simulink model "XMC_FFT2D_HDL_AIE"  (R2020a)
settings: Solver=FixedStepDiscrete  StartTime=0.0  StopTime=256*256*2  RelTol=1e-3
PreLoadFcn:
  | MRIDemo_PreloadFcn;
  | 
  | % configure hardware specifics information
  | clock_frequency = 150e6;
  | 
  | % corner bender info
  | clk = clock_frequency; %Hz
  | Tclk = 1/clk;
  | L2M = 8; % L2M=log2(M)
  | L2N = 8; % L2N=log2(N)
  | M = 2^L2M;
  | N = 2^L2N;
  | SSR = 1;
InitFcn:
  | xlEvaluateHDLBlocks('XMC_FFT2D_HDL_AIE')
undefined symbols (not defined in the file): c, gray, S, vsva2197, xcvc1902
libraries: xbsIndex_r4 x132, ModelComposer x6, dspxfrm3 x2, dspsrcs4 x2
(part 1 of 2)
settings Model: PauseTimes=256*254  SnapshotBufferSize=1000  SnapshotInterval=1  Creator=mmi  LastModifiedBy=viswanad
settings DataIOCC: ReturnWorkspaceOutputs=off
settings DebuggingCC: ArithmeticOperatorsInVariantConditions=warning
settings SFSimCC: SimUseLocalCustomCode=off  CustomCodeUndefinedFunction=UseInterfaceOnly
settings RTWCC: RTWUseLocalCustomCode=off

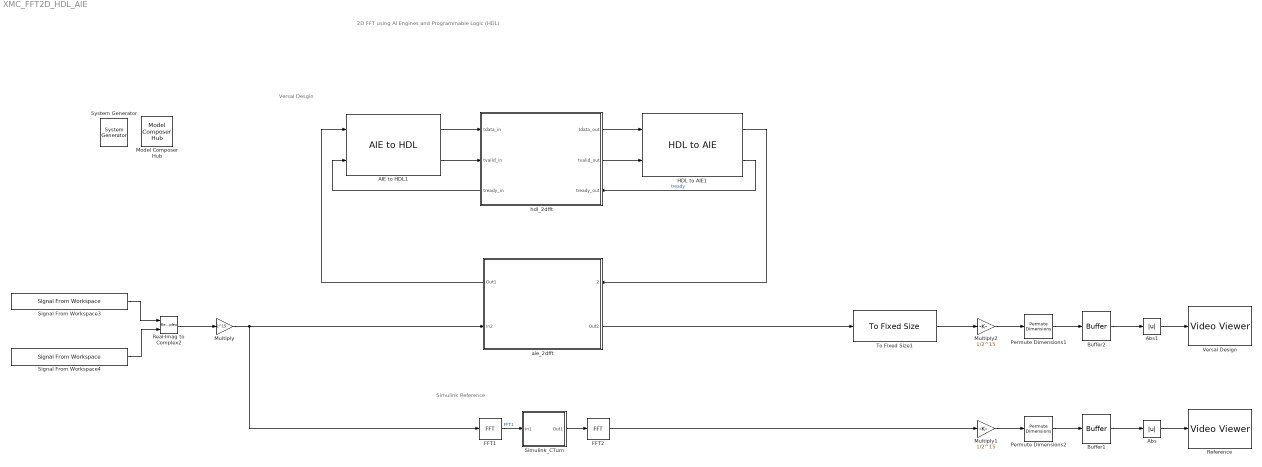
== system XMC_FFT2D_HDL_AIE ==
  note: Versal Desgin
  note: Simulink Reference
  note: 2D FFT using
      | AI Engines and Programmable Logic (HDL)
  " System Generator" : xbsIndex_r4/ System Generator  Tag=genX  xilinxfamily=versalaicore  part=xcvc1902  speed=-3HP-e-S  package=viva1596  synthesis_tool=Vivado  clock_wrapper=Clock Enables  directory=./netlist  proj_type=Vivado  Synth_file=Vivado Synthesis Defaults  Impl_file=Vivado Implementation Defaults  testbench=off  simulink_period=1  sysclk_period=4  dcm_input_clock_period=10  incr_netlist=off  trim_vbits=Everywhere in SubSystem  dbl_ovrd=According to Block Masks  core_generation=According to Block Masks  run_coregen=off  deprecated_control=off  eval_field=0  block_type=sysgen
  AIE to HDL1 : ModelComposer/AIE to HDL  OutDataType=uint32  OutSampleTime=1
      link override AIE to HDL_tready: inherit_from_input=on  hdl_port=on  rows=1  columns=1  UseAsDAC=off  DACChannel='1'  interface=None  automatic_assignment=on  address_offset=hex2dec('00')  intf_name=''  intf_description=''  timing_constraint=None  locs_specified=off  LOCs={}  io_standard={}
      link override AIE to HDL_tready: infoedit="Gateway out block.  Converts Xilinx fixed-point or floating-point type inputs into ouputs of type Simulink integer, single, double, or fixed-point.<br><br>Hardware notes:  In hardware these blocks become top level output ports or are discarded, depending on how they are configured."
  Abs : Abs
  Abs1 : Abs
  Buffer1 : Buffer  N=256  OutputFrames=off
  Buffer2 : Buffer  N=256  OutputFrames=off
  FFT1 : dspxfrm3/FFT  FFTImplementation=Auto  CompMethod=Table lookup  TableOpt=NEW  TableOptActive=Speed  BitRevOrder=off  Normalize=off  InheritFFTLength=on  FFTLength=64  WrapInput=on  roundingMode=Floor  overflowMode=off  firstCoeffDataTypeStr=Inherit: Same word length as input  firstCoeffLastDataTypeStr=Inherit: Same word length as input  prodOutputMode=Binary point scaling  prodOutputWordLength=32  prodOutputFracLength=0  prodOutputDataTypeStr=fixdt(1,32,0)  prodOutputLastDataTypeStr=fixdt(1,32,0)  accumMode=Binary point scaling  accumWordLength=48  accumFracLength=0  accumDataTypeStr=fixdt(1,48,0)  accumLastDataTypeStr=fixdt(1,48,0)  outputMode=Binary point scaling  outputWordLength=16  outputFracLength=0  outputDataTypeStr=fixdt(1,16,0)  outputMin=[]  outputMax=[]  outputLastDataTypeStr=fixdt(1,16,0)
  FFT2 : dspxfrm3/FFT  FFTImplementation=Auto  CompMethod=Table lookup  TableOpt=NEW  TableOptActive=Speed  BitRevOrder=off  Normalize=off  InheritFFTLength=on  FFTLength=64  WrapInput=on  roundingMode=Floor  overflowMode=off  firstCoeffDataTypeStr=Inherit: Same word length as input  firstCoeffLastDataTypeStr=Inherit: Same word length as input  prodOutputMode=Binary point scaling  prodOutputWordLength=32  prodOutputFracLength=0  prodOutputDataTypeStr=fixdt(1,32,0)  prodOutputLastDataTypeStr=fixdt(1,32,0)  accumMode=Binary point scaling  accumWordLength=48  accumFracLength=0  accumDataTypeStr=fixdt(1,48,0)  accumLastDataTypeStr=fixdt(1,48,0)  outputMode=Binary point scaling  outputWordLength=16  outputFracLength=0  outputDataTypeStr=fixdt(1,16,0)  outputMin=[]  outputMax=[]  outputLastDataTypeStr=fixdt(1,16,0)
  HDL to AIE1 : ModelComposer/HDL to AIE  OutDataType=int16 (c)  OutSampleTime=1  SamplesPerFrame=256  TreadySampleTime=1
  Model Composer Hub : ModelComposer/Model Composer Hub  CodeGeneration=off  SubsystemName=aie_2dfft  TargetDirectory=./code  ExportType=AI Engines  IpVendor=xilinx.com  IpLibrary=hls  IpVersion=1.0  IpHWLanguage=Verilog  AieCompilerOptions={}  CreateTestbench=on  TestbenchStackSize=10  RunAieSim=on  AieSimTimeout=50000  RunAieSimProfiling=off  LaunchVitisAnalyzer=off  PlotOutput=off  RunX86Sim=off  X86SimTimeout=10  PlatformType=Not Specified  ProjDevice=xcvc1902-vsva2197-2MP-e-S  ProjDevicePart=xcvc1902-vsva2197-2MP-e-S  SamplePeriod=-1  ClockFrequency=150  DataPathParallelism=1
  Multiply : Gain  Gain=2^15  OutDataTypeStr=int16
  Multiply1 : Gain  Gain=1/2^15  OutDataTypeStr=single
  Multiply2 : Gain  Gain=1/2^15  OutDataTypeStr=single
  Permute Dimensions1 : PermuteDimensions
  Permute Dimensions2 : PermuteDimensions
  Real-Imag to Complex2 : RealImagToComplex
  Reference : VideoViewer  Description=Simulink MRI Display  colormapValue=gray(256)  FigPos=[1258 828 663 270]
  Signal From Workspace3 : dspsrcs4/Signal From Workspace  X=MRIDemo_data_real_channel  Ts=1  nsamps=256  OutputAfterFinalValue=Setting to zero  ignoreOrWarnInputAndFrameLengths=off  OutputFrames=off
  Signal From Workspace4 : dspsrcs4/Signal From Workspace  X=MRIDemo_data_imag_channel  Ts=1  nsamps=256  OutputAfterFinalValue=Setting to zero  ignoreOrWarnInputAndFrameLengths=off  OutputFrames=off
  Simulink_CTurn : Subsystem
  To Fixed Size1 : ModelComposer/To Fixed Size  OutputSize=256  HasStatusOutput=off
  Versal Design : VideoViewer  Description=Simulink MRI Display  colormapValue=gray(256)  FigPos=[720 707 653 277]
  aie_2dfft : Subsystem
      settings: PortSchema="{\"entries\":[{\"content\":{\"sides\":[{\"content\":{\"connectorIds\":[\"Out2\",\"In1\"]},\"type\":\"ConnectorPlacement.EquallySpacedRectSide\",\"uuid\":\"ba116f73-e116-40b3-b2e5-304cba4df7e1\"},{\"content\":{\"connectorIds\":[\"In2\",\"Out1\"],\"side\":\"RIGHT\"},\"type\":\"ConnectorPlacement.EquallySpacedRectSide\",\"uuid\":\"f8ace37c-ffb0-4f56-a1b3-7eeef7565cfd\"},{\"content\":{\"connectorIds\":[],\"side\":\"TOP\"},\"type\":\"ConnectorPlacement.EquallySpacedRectSide\",\"uuid\":\"698d2e0a-1e8b-402b-bc99-cd34e1f9cd41\"}]},\"type\":\"ConnectorPlacement.EquallySpacedConnector\",\"uuid\":\"c9271cff-0d68-4ac4-bc57-5327e013a37e\"}],\"packageUris\":[\"http://schema.mathworks.com/mf0/Connector/R2020b\"],\"version\":\"1.0\"}"
  hdl_2dfft : Subsystem
      settings: PortSchema="{\"entries\":[{\"content\":{\"sides\":[{\"content\":{\"connectorIds\":[\"In1\",\"In2\",\"Out3\"]},\"type\":\"ConnectorPlacement.EquallySpacedRectSide\",\"uuid\":\"096cfc4a-45cf-495e-9dad-5ec39c034de1\"},{\"content\":{\"connectorIds\":[\"Out1\",\"Out2\",\"In3\"],\"side\":\"RIGHT\"},\"type\":\"ConnectorPlacement.EquallySpacedRectSide\",\"uuid\":\"c2f58c53-17c1-4e0f-8fe6-4ca31b4ae7e7\"},{\"content\":{\"connectorIds\":[],\"side\":\"TOP\"},\"type\":\"ConnectorPlacement.EquallySpacedRectSide\",\"uuid\":\"fc0a0e48-62d9-4bc4-85b8-28883543f418\"}]},\"type\":\"ConnectorPlacement.EquallySpacedConnector\",\"uuid\":\"4d40c623-5fa9-4077-a912-8400e8a8f04d\"}],\"packageUris\":[\"http://schema.mathworks.com/mf0/Connector/R2020b\"],\"version\":\"1.0\"}"
  wires:
  HDL to AIE1/1 -> aie_2dfft/2(" ")
  Real-Imag to Complex2/1 -> Multiply/1
  Signal From Workspace3/1 -> Real-Imag to Complex2/1
  Signal From Workspace4/1 -> Real-Imag to Complex2/2
  hdl_2dfft/2(tvalid_out) -> HDL to AIE1/2
  hdl_2dfft/1(tdata_out) -> HDL to AIE1/1
  AIE to HDL1/2 -> hdl_2dfft/2(tvalid_in)
  AIE to HDL1/1 -> hdl_2dfft/1(tdata_in)
  aie_2dfft/2(Out1) -> AIE to HDL1/1
  HDL to AIE1/2 -> hdl_2dfft/3(tready_out)  "tready"
  hdl_2dfft/3(tready_in) -> AIE to HDL1/2
  Multiply1/1 -> Permute Dimensions2/1
  Abs/1 -> Reference/1
  Permute Dimensions2/1 -> Buffer1/1
  Buffer1/1 -> Abs/1
  Multiply/1 -> FFT1/1, aie_2dfft/1(In2)
  FFT1/1 -> Simulink_CTurn/1(In1)  "FFT1"
  FFT2/1 -> Multiply1/1
  Simulink_CTurn/1(Out1) -> FFT2/1
  Abs1/1 -> Versal Design/1
  Buffer2/1 -> Abs1/1
  Permute Dimensions1/1 -> Buffer2/1
  Multiply2/1 -> Permute Dimensions1/1
  aie_2dfft/1(Out2) -> To Fixed Size1/1
  To Fixed Size1/1 -> Multiply2/1

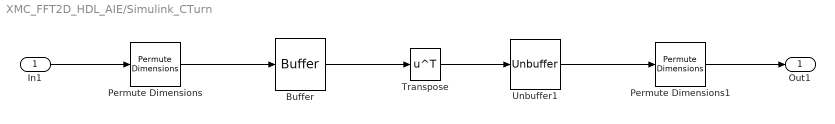
== system XMC_FFT2D_HDL_AIE/Simulink_CTurn ==
  In1 : Inport
  Buffer : Buffer  N=256  OutputFrames=off
  Permute Dimensions : PermuteDimensions
  Permute Dimensions1 : PermuteDimensions
  Transpose : Math  Operator=transpose  SignedPower=on  SaturateOnIntegerOverflow=on
  Unbuffer1 : Unbuffer
  Out1 : Outport  VectorParamsAs1DForOutWhenUnconnected=off
  wires:
  Permute Dimensions/1 -> Buffer/1
  Transpose/1 -> Unbuffer1/1
  Buffer/1 -> Transpose/1
  In1/1 -> Permute Dimensions/1
  Unbuffer1/1 -> Permute Dimensions1/1
  Permute Dimensions1/1 -> Out1/1

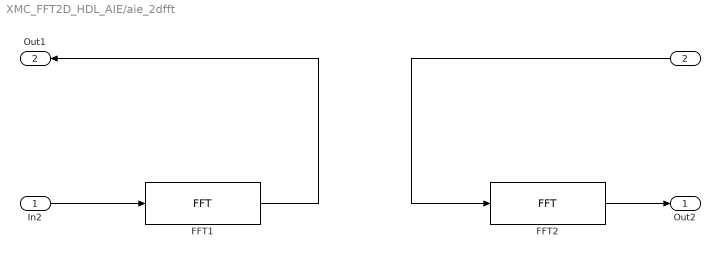
== system XMC_FFT2D_HDL_AIE/aie_2dfft ==
  In2 : Inport
  " " : Inport  Port=2
  FFT1 : ModelComposer/FFT  data_type=cint16  point_size=256  casc_length=1  shift_val=0  spec=meta_data_hl_fft.json
  FFT2 : ModelComposer/FFT  data_type=cint16  point_size=256  casc_length=1  shift_val=0  spec=meta_data_hl_fft.json
  Out2 : Outport
  Out1 : Outport  Port=2
  wires:
  FFT2/1 -> Out2/1
  " "/1 -> FFT2/1
  FFT1/1 -> Out1/1
  In2/1 -> FFT1/1

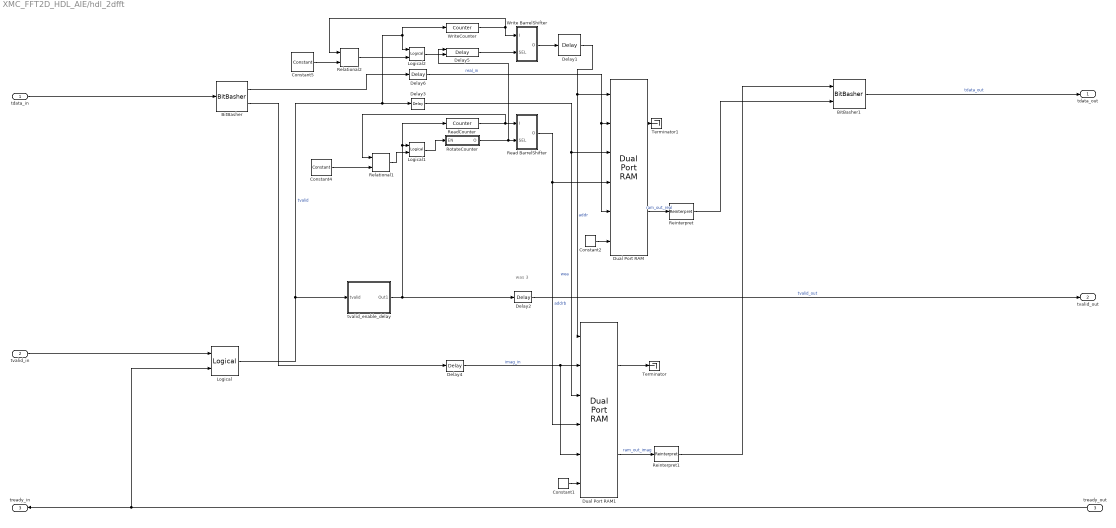
== system XMC_FFT2D_HDL_AIE/hdl_2dfft ==
  note: was 3
  tdata_in : Inport
  tvalid_in : Inport  Port=2
  tready_out : Inport  Port=3
  BitBasher : xbsIndex_r4/BitBasher  bitexpr=|  display_expr=off  sr_1=re  arith_type1="Signed  (2's comp)"  bin_pt1=0  sr_2=im  arith_type2="Signed  (2's comp)"  bin_pt2=0  sr_3=3  arith_type3=Unsigned  bin_pt3=0  sr_4=4  arith_type4=Unsigned  bin_pt4=0  dbl_ovrd=off  block_type=bitbasher
      | re={cplx_in[15:0]};
      | im={cplx_in[31:16]};
  BitBasher1 : xbsIndex_r4/BitBasher  bitexpr=cplx_out={im[15:0], re[15:0]};  display_expr=off  sr_1=cplx_out  arith_type1=Unsigned  bin_pt1=0  sr_2=im  arith_type2=Unsigned  bin_pt2=0  sr_3=3  arith_type3=Unsigned  bin_pt3=0  sr_4=4  arith_type4=Unsigned  bin_pt4=0  dbl_ovrd=off  block_type=bitbasher
  Constant1 : xbsIndex_r4/Constant  const=0  gui_display_data_type=Boolean  arith_type=Boolean  n_bits=40  bin_pt=20  preci_type=Single  exp_width=8  frac_width=24  explicit_period=off  period=1  equ=P=C  opselect=C  inp2=PCIN>>17  opr=+  inp1=P  carry=CIN  dbl_ovrd=off  block_type=constant
  Constant2 : xbsIndex_r4/Constant  const=0  gui_display_data_type=Boolean  arith_type=Boolean  n_bits=40  bin_pt=20  preci_type=Single  exp_width=8  frac_width=24  explicit_period=off  period=1  equ=P=C  opselect=C  inp2=PCIN>>17  opr=+  inp1=P  carry=CIN  dbl_ovrd=off  block_type=constant
  Constant4 : xbsIndex_r4/Constant  const=2^(L2M+L2N)-1  gui_display_data_type=Fixed-point  arith_type=Unsigned  n_bits=L2M+L2N  bin_pt=0  preci_type=Single  exp_width=8  frac_width=24  explicit_period=off  period=1  equ=P=C  opselect=C  inp2=PCIN>>17  opr=+  inp1=P  carry=CIN  dbl_ovrd=off  block_type=constant
  Constant5 : xbsIndex_r4/Constant  const=2^(L2M+L2N)-1  gui_display_data_type=Fixed-point  arith_type=Unsigned  n_bits=L2M+L2N  bin_pt=0  preci_type=Single  exp_width=8  frac_width=24  explicit_period=off  period=1  equ=P=C  opselect=C  inp2=PCIN>>17  opr=+  inp1=P  carry=CIN  dbl_ovrd=off  block_type=constant
  Delay1 : xbsIndex_r4/Delay  rst=off  infoeditControl=Selection of Reset will increase slice count due to use of real FFs and instead of SRLs  en=off  latency=1  reg_retiming=off  dbl_ovrd=off  block_type=delay
  Delay2 : xbsIndex_r4/Delay  rst=off  infoeditControl=Selection of Reset will increase slice count due to use of real FFs and instead of SRLs  en=off  latency=3  reg_retiming=off  dbl_ovrd=off  block_type=delay
  Delay3 : xbsIndex_r4/Delay  rst=off  infoeditControl=Selection of Reset will increase slice count due to use of real FFs and instead of SRLs  en=off  latency=2  reg_retiming=off  dbl_ovrd=off  block_type=delay
  Delay4 : xbsIndex_r4/Delay  rst=off  infoeditControl=Selection of Reset will increase slice count due to use of real FFs and instead of SRLs  en=off  latency=2  reg_retiming=off  dbl_ovrd=off  block_type=delay
  Delay5 : xbsIndex_r4/Delay  rst=off  infoeditControl=Selection of Reset will increase slice count due to use of real FFs and instead of SRLs  en=on  latency=1  reg_retiming=off  dbl_ovrd=off  block_type=delay
  Delay6 : xbsIndex_r4/Delay  rst=off  infoeditControl=Selection of Reset will increase slice count due to use of real FFs and instead of SRLs  en=off  latency=2  reg_retiming=off  dbl_ovrd=off  block_type=delay
  Dual Port RAM : xbsIndex_r4/Dual Port RAM  depth=2^L2M*2^L2N  initVector=zeros(2^L2M*2^L2N,1)  distributed_mem=Block RAM  init_a=0  init_b=0  rst_a=off  rst_b=off  en_a=off  en_b=off  latency=2  write_mode_A=Read After Write  write_mode_B=Read After Write  optimize=Area  dbl_ovrd=off  simulation_type=fast_sim  block_type=dpram
  Dual Port RAM1 : xbsIndex_r4/Dual Port RAM  depth=2^L2M*2^L2N  initVector=zeros(2^L2M*2^L2N,1)  distributed_mem=Block RAM  init_a=0  init_b=0  rst_a=off  rst_b=off  en_a=off  en_b=off  latency=2  write_mode_A=Read After Write  write_mode_B=Read After Write  optimize=Area  dbl_ovrd=off  simulation_type=fast_sim  block_type=dpram
  Logical : xbsIndex_r4/Logical  logical_function=AND  inputs=2  en=off  latency=0  precision=Full  arith_type=Unsigned  n_bits=16  bin_pt=0  align_bp=on  dbl_ovrd=off  block_type=logical
  Logical1 : xbsIndex_r4/Logical  logical_function=AND  inputs=2  en=off  latency=0  precision=Full  arith_type=Unsigned  n_bits=16  bin_pt=0  align_bp=on  dbl_ovrd=off  block_type=logical
  Logical2 : xbsIndex_r4/Logical  logical_function=AND  inputs=2  en=off  latency=0  precision=Full  arith_type=Unsigned  n_bits=16  bin_pt=0  align_bp=on  dbl_ovrd=off  block_type=logical
  Read BarrelShifter : Subsystem  mask{barrel_length=L2M+L2N}
      mask prompts: barrel_length "Barrel Length"
      mask init:
      | %%%%%%%%%%%%%%%%%%%%%%%%%%%%%%%%%%%%%%%%%%%%%%%%%%%%%
      | % Parametric Barrel Shifter Mask Initialization Script
      | % 18DEC2017: Creation
      | %%%%%%%%%%%%%%%%%%%%%%%%%%%%%%%%%%%%%%%%%%%%%%%%%%%%%
      | this=gcb;
      | 
      | %%%%%%%%%%%%%%%%%%%%%%%%%%%%%%%%%%%%%%%%%%%%%%%%%%%%%
      | % Delete wires and certain blocks; retain IO ports so parent
      | % mask block will not require re-connection
      | %%%%%%%%%%%%%%%%%%%%%%%%%%%%%%%%%%%%%%%%%%%%%%%%%%%%%
      | 
      | % delete all blocks except for d1 and q1
      | allblocks = find_system(this, 'LookUnderMasks','on','SearchDepth',1);
      | 
      | ToKeep = {'I';'O';'SEL';'Mux';'RotateLeft1'};
      | 
      | %// add systemname to strings
      | ToKeep = strcat(repmat({[this  '/']},numel(ToKeep),1), ToKeep);
      | 
      | %// create mask
      | ToDelete = setdiff(allblocks,ToKeep);
      | %// filter out main system
      | ToDelete = setxor(ToDelete,this);
      | 
      | cellfun(@(x) delete_block(x),ToDelete)
      | 
      | % delete lines
      | L = find_system(this,'LookUnderMasks','on','SearchDepth',1,'FindAll','on','type','line');
      | delete_line(L(1:end));
      | 
      | %%%%%%%%%%%%%%%%%%%%%%%%%%%%%%%%%%%%%%%%%%%%%%%%%%%%%%
      | % instantiate RotateLeft blocks and configure
      | %%%%%%%%%%%%%%%%%%%%%%%%%%%%%%%%%%%%%%%%%%%%%%%%%%%%%%
      | blockName1 = strcat(this,'/RotateLeft1');
      | x_loc = 70;
      | y_loc = 70;
      | for i = 2:barrel_length-1
      |     blockName = strcat(this,'/RotateLeft',num2str(i));
      |     blockHandle = add_block(blockName1,blockName, 'position',[x_loc,y_loc,x_loc+60,y_loc+20], ...
      |         'NB',num2str(i));
      |     y_loc = y_loc + 40;
      | end
      | 
      | %%%%%%%%%%%%%%%%%%%%%%%%%%%%%%%%%%%%%%%%%%%%%%%%%%%%%%
      | % Set mux parameters
      | %%%%%%%%%%%%%%%%%%%%%%%%%%%%%%%%%%%%%%%%%%%%%%%%%%%%%%
      | 
      | myMux = strcat(this,'/Mux');
      | set_param(myMux, 'inputs', barrel_length-2);
      | 
      | %%%%%%%%%%%%%%%%%%%%%%%%%%%%%%%%%%%%%%%%%%%%%%%%%%%%%%
      | % wires
      | %%%%%%%%%%%%%%%%%%%%%%%%%%%%%%%%%%%%%%%%%%%%%%%%%%%%%%
      | 
      | % RotateLeft to mux
      | 
      | h_myMux = get_param(myMux,'PortHandles');
      | 
      | for i = 1:barrel_length-1  
      |   blockName = strcat(this,'/RotateLeft',num2str(i));
      |   h_RotateLeft =  get_param(blockName,'PortHandles');
      |   add_line(this,{h_RotateLeft.Outport} ,{h_myMux.Inport(i+2)},'autorouting','on');
      | end
      | 
      | % mux to outport
      | h_myOutport = get_param(strcat(this,'/O'), 'PortHandles');
      | 
      | add_line(this,{h_myMux.Outport} ,{h_myOutport.Inport},'autorouting','on');
      | 
      | % inport to RotateLeft
      | h_myInport = get_param(strcat(this,'/I'), 'PortHandles');
      | 
      | for i = 1:barrel_length-1  
      |   blockName = strcat(this,'/RotateLeft',num2str(i));
      |   h_RotateLeft =  get_param(blockName,'PortHandles');
      |   add_line(this,{h_myInport.Outport} ,{h_RotateLeft.Inport},'autorouting','on');
      | end
      | 
      | % inport to mux
      | add_line(this,{h_myInport.Outport} ,{h_myMux.Inport(2)},'autorouting','on');
      | 
      | % SEL to mux
      | h_mySEL = get_param(strcat(this,'/SEL'), 'PortHandles');
      | add_line(this,{h_mySEL.Outport} ,{h_myMux.Inport(1)},'autorouting','on');
  ReadCounter : xbsIndex_r4/Counter  cnt_type=Free Running  cnt_to=Inf  operation=Up  start_count=0  cnt_by_val=1  arith_type=Unsigned  n_bits=L2M+L2N  bin_pt=0  load_pin=off  rst=off  en=on  explicit_period=off  period=1  use_behavioral_HDL=off  implementation=Fabric  dbl_ovrd=off  block_type=counter
  Reinterpret : xbsIndex_r4/Reinterpret  force_arith_type=on  arith_type=Unsigned  force_bin_pt=off  bin_pt=0  block_type=reinterpret
  Reinterpret1 : xbsIndex_r4/Reinterpret  force_arith_type=on  arith_type=Unsigned  force_bin_pt=off  bin_pt=0  block_type=reinterpret
  Relational1 : xbsIndex_r4/Relational  mode=a=b  op_type=Bool  en=off  latency=0  dbl_ovrd=off  block_type=relational
  Relational2 : xbsIndex_r4/Relational  mode=a=b  op_type=Bool  en=off  latency=0  dbl_ovrd=off  block_type=relational
  RotateCounter : Subsystem  mask{L2M=L2M, L2N=L2N}
  Terminator : Terminator
  Terminator1 : Terminator
  Write BarrelShifter : Subsystem  mask{barrel_length=L2M+L2N}
      mask prompts: barrel_length "Barrel Length"
      mask init: same as XMC_FFT2D_HDL_AIE/hdl_2dfft/Read BarrelShifter
  WriteCounter : xbsIndex_r4/Counter  cnt_type=Free Running  cnt_to=Inf  operation=Up  start_count=0  cnt_by_val=1  arith_type=Unsigned  n_bits=L2M+L2N  bin_pt=0  load_pin=off  rst=off  en=on  explicit_period=off  period=1  use_behavioral_HDL=off  implementation=Fabric  dbl_ovrd=off  block_type=counter
  tvalid_enable_delay : Subsystem
  tdata_out : Outport
  tvalid_out : Outport  Port=2
  tready_in : Outport  Port=3
  wires:
  Constant4/1 -> Relational1/2
  RotateCounter/1(O) -> Delay5/1, Read BarrelShifter/2(SEL)
  Constant1/1 -> Dual Port RAM1/6
  Reinterpret/1 -> BitBasher1/2
  Delay5/1 -> Write BarrelShifter/2(SEL)
  Relational1/1 -> Logical1/2
  Logical2/1 -> Delay5/2
  Constant5/1 -> Relational2/2
  ReadCounter/1 -> Read BarrelShifter/1(I), Relational1/1
  Dual Port RAM/2 -> Reinterpret/1  "ram_out_real"
  Read BarrelShifter/1(O) -> Dual Port RAM/4, Dual Port RAM1/4  "addrb"
  WriteCounter/1 -> Write BarrelShifter/1(I), Relational2/1
  Logical1/1 -> RotateCounter/1(EN)
  Delay4/1 -> Dual Port RAM1/5, Dual Port RAM1/2  "imag_in"
  BitBasher/2 -> Delay4/1
  Delay6/1 -> Dual Port RAM/5, Dual Port RAM/2  "real_in"
  tdata_in/1 -> BitBasher/1
  Delay3/1 -> Dual Port RAM1/3, Dual Port RAM/3  "wea"
  Delay2/1 -> tvalid_out/1  "tvalid_out"
  Dual Port RAM/1 -> Terminator1/1
  BitBasher1/1 -> tdata_out/1  "tdata_out"
  Logical/1 -> Logical2/1, WriteCounter/1, Delay3/1, tvalid_enable_delay/1(tvalid)  "tvalid"
  Constant2/1 -> Dual Port RAM/6
  Dual Port RAM1/1 -> Terminator/1
  Write BarrelShifter/1(O) -> Delay1/1
  tvalid_in/1 -> Logical/1
  Relational2/1 -> Logical2/2
  Reinterpret1/1 -> BitBasher1/1
  tvalid_enable_delay/1(Out1) -> Delay2/1, ReadCounter/1, Logical1/1
  BitBasher/1 -> Delay6/1
  Delay1/1 -> Dual Port RAM/1, Dual Port RAM1/1  "addr"
  Dual Port RAM1/2 -> Reinterpret1/1  "ram_out_imag"
  tready_out/1 -> Logical/2, tready_in/1

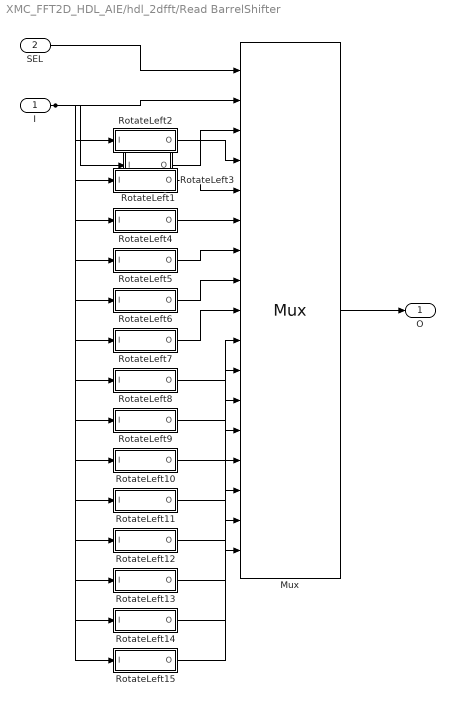
== system XMC_FFT2D_HDL_AIE/hdl_2dfft/Read BarrelShifter ==
  I : Inport
  SEL : Inport  Port=2
  Mux : xbsIndex_r4/Mux  inputs=16  en=off  latency=1  precision=Full  arith_type=Unsigned  n_bits=16  bin_pt=14  quantization=Truncate  overflow=Wrap  dbl_ovrd=off  block_type=mux
  RotateLeft1 : Subsystem  mask{NB=1, W=barrel_length}
      mask prompts: NB "Number of bits (cannot be 0):"; W "Width"
  RotateLeft10 : Subsystem  mask{NB=10, W=barrel_length}
      mask prompts: NB "Number of bits (cannot be 0):"; W "Width"
  RotateLeft11 : Subsystem  mask{NB=11, W=barrel_length}
      mask prompts: NB "Number of bits (cannot be 0):"; W "Width"
  RotateLeft12 : Subsystem  mask{NB=12, W=barrel_length}
      mask prompts: NB "Number of bits (cannot be 0):"; W "Width"
  RotateLeft13 : Subsystem  mask{NB=13, W=barrel_length}
      mask prompts: NB "Number of bits (cannot be 0):"; W "Width"
  RotateLeft14 : Subsystem  mask{NB=14, W=barrel_length}
      mask prompts: NB "Number of bits (cannot be 0):"; W "Width"
  RotateLeft15 : Subsystem  mask{NB=15, W=barrel_length}
      mask prompts: NB "Number of bits (cannot be 0):"; W "Width"
  RotateLeft2 : Subsystem  mask{NB=2, W=barrel_length}
      mask prompts: NB "Number of bits (cannot be 0):"; W "Width"
  RotateLeft3 : Subsystem  mask{NB=3, W=barrel_length}
      mask prompts: NB "Number of bits (cannot be 0):"; W "Width"
  RotateLeft4 : Subsystem  mask{NB=4, W=barrel_length}
      mask prompts: NB "Number of bits (cannot be 0):"; W "Width"
  RotateLeft5 : Subsystem  mask{NB=5, W=barrel_length}
      mask prompts: NB "Number of bits (cannot be 0):"; W "Width"
  RotateLeft6 : Subsystem  mask{NB=6, W=barrel_length}
      mask prompts: NB "Number of bits (cannot be 0):"; W "Width"
  RotateLeft7 : Subsystem  mask{NB=7, W=barrel_length}
      mask prompts: NB "Number of bits (cannot be 0):"; W "Width"
  RotateLeft8 : Subsystem  mask{NB=8, W=barrel_length}
      mask prompts: NB "Number of bits (cannot be 0):"; W "Width"
  RotateLeft9 : Subsystem  mask{NB=9, W=barrel_length}
      mask prompts: NB "Number of bits (cannot be 0):"; W "Width"
  O : Outport
  wires:
  RotateLeft1/1(O) -> Mux/3
  RotateLeft2/1(O) -> Mux/4
  RotateLeft3/1(O) -> Mux/5
  RotateLeft4/1(O) -> Mux/6
  RotateLeft5/1(O) -> Mux/7
  RotateLeft6/1(O) -> Mux/8
  RotateLeft7/1(O) -> Mux/9
  RotateLeft8/1(O) -> Mux/10
  RotateLeft9/1(O) -> Mux/11
  RotateLeft10/1(O) -> Mux/12
  RotateLeft11/1(O) -> Mux/13
  RotateLeft12/1(O) -> Mux/14
  RotateLeft13/1(O) -> Mux/15
  RotateLeft14/1(O) -> Mux/16
  RotateLeft15/1(O) -> Mux/17
  Mux/1 -> O/1
  I/1 -> RotateLeft1/1(I), RotateLeft2/1(I), RotateLeft3/1(I), RotateLeft4/1(I), RotateLeft5/1(I), RotateLeft6/1(I), RotateLeft7/1(I), RotateLeft8/1(I), RotateLeft9/1(I), RotateLeft10/1(I), RotateLeft11/1(I), RotateLeft12/1(I), RotateLeft13/1(I), RotateLeft14/1(I), RotateLeft15/1(I), Mux/2
  SEL/1 -> Mux/1

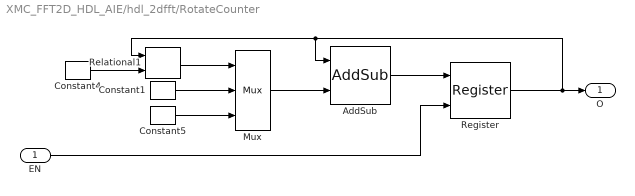
== system XMC_FFT2D_HDL_AIE/hdl_2dfft/RotateCounter ==
  EN : Inport
  AddSub : xbsIndex_r4/AddSub  mode=Addition  use_carryin=off  use_carryout=off  en=off  latency=0  precision=User Defined  arith_type=Unsigned  n_bits=ceil(log2(L2M+L2N))  bin_pt=0  quantization=Truncate  overflow=Wrap  use_behavioral_HDL=off  hw_selection=Fabric  pipelined=off  dbl_ovrd=off  block_type=addsub
  Constant1 : xbsIndex_r4/Constant  const=L2N  gui_display_data_type=Fixed-point  arith_type=Unsigned  n_bits=ceil(log2(L2M+L2N))  bin_pt=0  preci_type=Single  exp_width=8  frac_width=24  explicit_period=on  period=1  equ=P=C  opselect=C  inp2=PCIN>>17  opr=+  inp1=P  carry=CIN  dbl_ovrd=off  block_type=constant
  Constant4 : xbsIndex_r4/Constant  const=L2M  gui_display_data_type=Fixed-point  arith_type=Unsigned  n_bits=ceil(log2(L2M+L2N))  bin_pt=0  preci_type=Single  exp_width=8  frac_width=24  explicit_period=on  period=1  equ=P=C  opselect=C  inp2=PCIN>>17  opr=+  inp1=P  carry=CIN  dbl_ovrd=off  block_type=constant
  Constant5 : xbsIndex_r4/Constant  const=2^ceil(log2(L2M+L2N))-L2M  gui_display_data_type=Fixed-point  arith_type=Unsigned  n_bits=ceil(log2(L2M+L2N))  bin_pt=0  preci_type=Single  exp_width=8  frac_width=24  explicit_period=on  period=1  equ=P=C  opselect=C  inp2=PCIN>>17  opr=+  inp1=P  carry=CIN  dbl_ovrd=off  block_type=constant
  Mux : xbsIndex_r4/Mux  inputs=2  en=off  latency=0  precision=Full  arith_type=Unsigned  n_bits=16  bin_pt=14  quantization=Truncate  overflow=Wrap  dbl_ovrd=off  block_type=mux
  Register : xbsIndex_r4/Register  init=L2N  rst=off  en=on  dbl_ovrd=off  block_type=register
  Relational1 : xbsIndex_r4/Relational  mode=a>=b  op_type=Bool  en=off  latency=0  dbl_ovrd=off  block_type=relational
  O : Outport
  wires:
  EN/1 -> Register/2
  Constant4/1 -> Relational1/2
  AddSub/1 -> Register/1
  Constant5/1 -> Mux/3
  Constant1/1 -> Mux/2
  Mux/1 -> AddSub/2
  Relational1/1 -> Mux/1
  Register/1 -> Relational1/1, AddSub/1, O/1

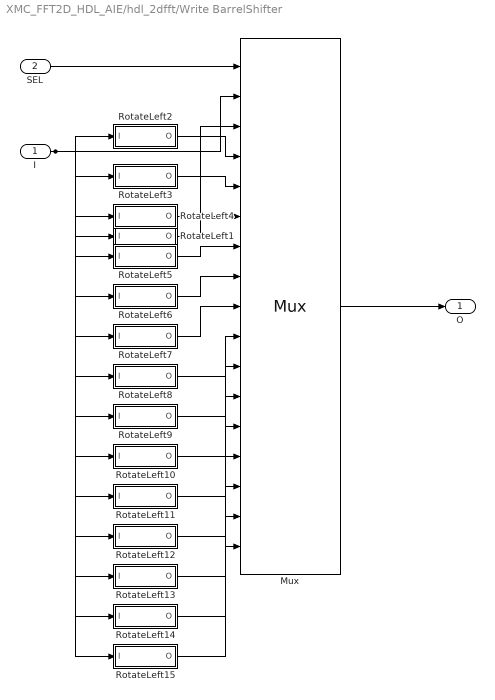
== system XMC_FFT2D_HDL_AIE/hdl_2dfft/Write BarrelShifter ==
  I : Inport
  SEL : Inport  Port=2
  Mux : xbsIndex_r4/Mux  inputs=16  en=off  latency=1  precision=Full  arith_type=Unsigned  n_bits=16  bin_pt=14  quantization=Truncate  overflow=Wrap  dbl_ovrd=off  block_type=mux
  RotateLeft1 : Subsystem  mask{NB=1, W=barrel_length}
      mask prompts: NB "Number of bits (cannot be 0):"; W "Width"
  RotateLeft10 : Subsystem  mask{NB=10, W=barrel_length}
      mask prompts: NB "Number of bits (cannot be 0):"; W "Width"
  RotateLeft11 : Subsystem  mask{NB=11, W=barrel_length}
      mask prompts: NB "Number of bits (cannot be 0):"; W "Width"
  RotateLeft12 : Subsystem  mask{NB=12, W=barrel_length}
      mask prompts: NB "Number of bits (cannot be 0):"; W "Width"
  RotateLeft13 : Subsystem  mask{NB=13, W=barrel_length}
      mask prompts: NB "Number of bits (cannot be 0):"; W "Width"
  RotateLeft14 : Subsystem  mask{NB=14, W=barrel_length}
      mask prompts: NB "Number of bits (cannot be 0):"; W "Width"
  RotateLeft15 : Subsystem  mask{NB=15, W=barrel_length}
      mask prompts: NB "Number of bits (cannot be 0):"; W "Width"
  RotateLeft2 : Subsystem  mask{NB=2, W=barrel_length}
      mask prompts: NB "Number of bits (cannot be 0):"; W "Width"
  RotateLeft3 : Subsystem  mask{NB=3, W=barrel_length}
      mask prompts: NB "Number of bits (cannot be 0):"; W "Width"
  RotateLeft4 : Subsystem  mask{NB=4, W=barrel_length}
      mask prompts: NB "Number of bits (cannot be 0):"; W "Width"
  RotateLeft5 : Subsystem  mask{NB=5, W=barrel_length}
      mask prompts: NB "Number of bits (cannot be 0):"; W "Width"
  RotateLeft6 : Subsystem  mask{NB=6, W=barrel_length}
      mask prompts: NB "Number of bits (cannot be 0):"; W "Width"
  RotateLeft7 : Subsystem  mask{NB=7, W=barrel_length}
      mask prompts: NB "Number of bits (cannot be 0):"; W "Width"
  RotateLeft8 : Subsystem  mask{NB=8, W=barrel_length}
      mask prompts: NB "Number of bits (cannot be 0):"; W "Width"
  RotateLeft9 : Subsystem  mask{NB=9, W=barrel_length}
      mask prompts: NB "Number of bits (cannot be 0):"; W "Width"
  O : Outport
  wires:
  RotateLeft1/1(O) -> Mux/3
  RotateLeft2/1(O) -> Mux/4
  RotateLeft3/1(O) -> Mux/5
  RotateLeft4/1(O) -> Mux/6
  RotateLeft5/1(O) -> Mux/7
  RotateLeft6/1(O) -> Mux/8
  RotateLeft7/1(O) -> Mux/9
  RotateLeft8/1(O) -> Mux/10
  RotateLeft9/1(O) -> Mux/11
  RotateLeft10/1(O) -> Mux/12
  RotateLeft11/1(O) -> Mux/13
  RotateLeft12/1(O) -> Mux/14
  RotateLeft13/1(O) -> Mux/15
  RotateLeft14/1(O) -> Mux/16
  RotateLeft15/1(O) -> Mux/17
  Mux/1 -> O/1
  I/1 -> RotateLeft1/1(I), RotateLeft2/1(I), RotateLeft3/1(I), RotateLeft4/1(I), RotateLeft5/1(I), RotateLeft6/1(I), RotateLeft7/1(I), RotateLeft8/1(I), RotateLeft9/1(I), RotateLeft10/1(I), RotateLeft11/1(I), RotateLeft12/1(I), RotateLeft13/1(I), RotateLeft14/1(I), RotateLeft15/1(I), Mux/2
  SEL/1 -> Mux/1

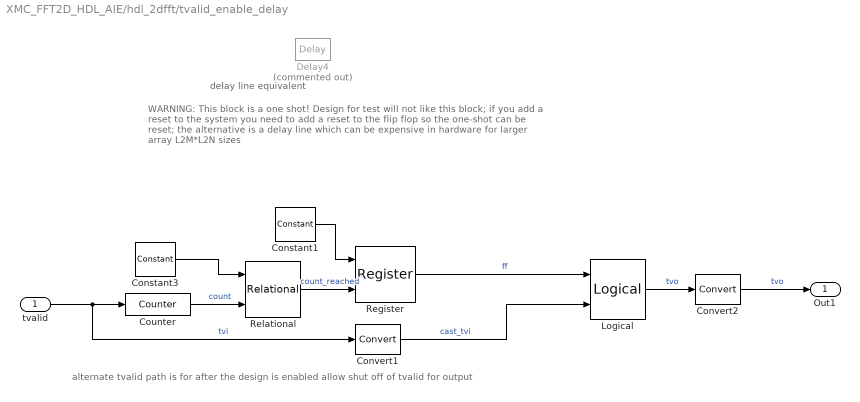
== system XMC_FFT2D_HDL_AIE/hdl_2dfft/tvalid_enable_delay ==
  note: alternate tvalid path is for after the design is enabled allow shut off of tvalid for output
  note: delay line equivalent
  note: WARNING: This block is a one shot! Design for test will not like this block; if you add a reset to the system you need to add a reset to the flip flop so the one-shot can be reset; the alternative is a delay line which can be expensive in hardware for larger array L2M*L2N sizes
  tvalid : Inport
  Constant1 : xbsIndex_r4/Constant  const=1  gui_display_data_type=Fixed-point  arith_type=Unsigned  n_bits=1  bin_pt=0  preci_type=Single  exp_width=8  frac_width=24  explicit_period=off  period=1  equ=P=C  opselect=C  inp2=PCIN>>17  opr=+  inp1=P  carry=CIN  dbl_ovrd=off  block_type=constant
  Constant3 : xbsIndex_r4/Constant  const=2^(L2M+L2N)-(2^L2M+2^L2N)+1  gui_display_data_type=Fixed-point  arith_type=Unsigned  n_bits=L2M+L2N  bin_pt=0  preci_type=Single  exp_width=8  frac_width=24  explicit_period=off  period=1  equ=P=C  opselect=C  inp2=PCIN>>17  opr=+  inp1=P  carry=CIN  dbl_ovrd=off  block_type=constant
  Convert1 : xbsIndex_r4/Convert  gui_display_data_type=Fixed-point  arith_type=Unsigned  n_bits=1  bin_pt=0  float_type=Single  exp_bits=8  fraction_bits=24  quantization=Truncate  overflow=Wrap  en=off  latency=0  pipeline=off  dbl_ovrd=off  block_type=convert
  Convert2 : xbsIndex_r4/Convert  gui_display_data_type=Boolean  arith_type=Boolean  n_bits=1  bin_pt=0  float_type=Single  exp_bits=8  fraction_bits=24  quantization=Truncate  overflow=Wrap  en=off  latency=0  pipeline=off  dbl_ovrd=off  block_type=convert
  Counter : xbsIndex_r4/Counter  cnt_type=Count Limited  cnt_to=2^(L2M+L2N)-(2^L2M+2^L2N)+2  operation=Up  start_count=0  cnt_by_val=1  arith_type=Unsigned  n_bits=L2M+L2N  bin_pt=0  load_pin=off  rst=off  en=on  explicit_period=on  period=1  use_behavioral_HDL=off  implementation=Fabric  dbl_ovrd=off  block_type=counter
  Delay4 : xbsIndex_r4/Delay  Commented=on  rst=off  infoeditControl=Selection of Reset will increase slice count due to use of real FFs and instead of SRLs  en=off  latency=2^(L2M+L2N)-(2^L2M+2^L2N)+2  reg_retiming=off  dbl_ovrd=off  block_type=delay
  Logical : xbsIndex_r4/Logical  logical_function=AND  inputs=2  en=off  latency=1  precision=Full  arith_type=Unsigned  n_bits=16  bin_pt=0  align_bp=on  dbl_ovrd=off  block_type=logical
  Register : xbsIndex_r4/Register  init=0  rst=off  en=on  dbl_ovrd=off  block_type=register
  Relational : xbsIndex_r4/Relational  mode=a=b  op_type=Bool  en=off  latency=0  dbl_ovrd=off  block_type=relational
  Out1 : Outport
  wires:
  Register/1 -> Logical/1  "ff"
  tvalid/1 -> Counter/1, Convert1/1  "tvi"
  Counter/1 -> Relational/2  "count"
  Relational/1 -> Register/2  "count_reached"
  Convert2/1 -> Out1/1  "tvo"
  Constant3/1 -> Relational/1
  Convert1/1 -> Logical/2  "cast_tvi"
  Constant1/1 -> Register/1
  Logical/1 -> Convert2/1  "tvo"

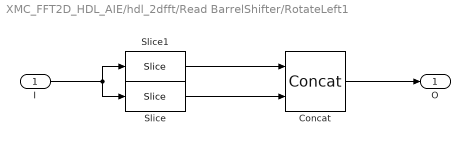
== system XMC_FFT2D_HDL_AIE/hdl_2dfft/Read BarrelShifter/RotateLeft1 ==
  I : Inport
  Concat : xbsIndex_r4/Concat  num_inputs=2  dbl_ovrd=off  block_type=concat
  Slice : xbsIndex_r4/Slice  nbits=NB  boolean_output=off  mode=Upper Bit Location + Width  bit1=0  base1=MSB of Input  bit0=0  base0=LSB of Input  dbl_ovrd=off  block_type=slice
  Slice1 : xbsIndex_r4/Slice  nbits=W-NB  boolean_output=off  mode=Lower Bit Location + Width  bit1=0  base1=MSB of Input  bit0=0  base0=LSB of Input  dbl_ovrd=off  block_type=slice
  O : Outport
  wires:
  Slice1/1 -> Concat/1
  Slice/1 -> Concat/2
  Concat/1 -> O/1
  I/1 -> Slice/1, Slice1/1

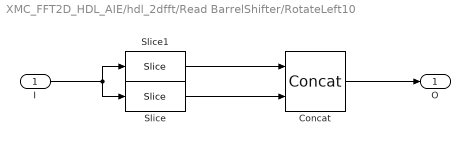
== system XMC_FFT2D_HDL_AIE/hdl_2dfft/Read BarrelShifter/RotateLeft10 ==
  I : Inport
  Concat : xbsIndex_r4/Concat  num_inputs=2  dbl_ovrd=off  block_type=concat
  Slice : xbsIndex_r4/Slice  nbits=NB  boolean_output=off  mode=Upper Bit Location + Width  bit1=0  base1=MSB of Input  bit0=0  base0=LSB of Input  dbl_ovrd=off  block_type=slice
  Slice1 : xbsIndex_r4/Slice  nbits=W-NB  boolean_output=off  mode=Lower Bit Location + Width  bit1=0  base1=MSB of Input  bit0=0  base0=LSB of Input  dbl_ovrd=off  block_type=slice
  O : Outport
  wires:
  I/1 -> Slice1/1, Slice/1
  Concat/1 -> O/1
  Slice/1 -> Concat/2
  Slice1/1 -> Concat/1

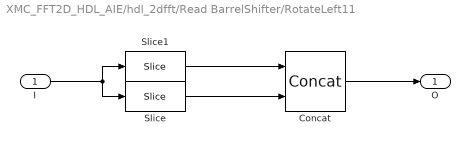
== system XMC_FFT2D_HDL_AIE/hdl_2dfft/Read BarrelShifter/RotateLeft11 ==
  I : Inport
  Concat : xbsIndex_r4/Concat  num_inputs=2  dbl_ovrd=off  block_type=concat
  Slice : xbsIndex_r4/Slice  nbits=NB  boolean_output=off  mode=Upper Bit Location + Width  bit1=0  base1=MSB of Input  bit0=0  base0=LSB of Input  dbl_ovrd=off  block_type=slice
  Slice1 : xbsIndex_r4/Slice  nbits=W-NB  boolean_output=off  mode=Lower Bit Location + Width  bit1=0  base1=MSB of Input  bit0=0  base0=LSB of Input  dbl_ovrd=off  block_type=slice
  O : Outport
  wires:
  I/1 -> Slice1/1, Slice/1
  Concat/1 -> O/1
  Slice/1 -> Concat/2
  Slice1/1 -> Concat/1

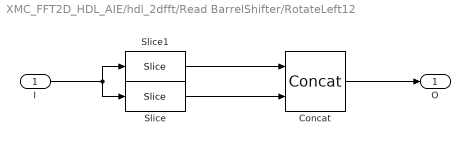
== system XMC_FFT2D_HDL_AIE/hdl_2dfft/Read BarrelShifter/RotateLeft12 ==
  I : Inport
  Concat : xbsIndex_r4/Concat  num_inputs=2  dbl_ovrd=off  block_type=concat
  Slice : xbsIndex_r4/Slice  nbits=NB  boolean_output=off  mode=Upper Bit Location + Width  bit1=0  base1=MSB of Input  bit0=0  base0=LSB of Input  dbl_ovrd=off  block_type=slice
  Slice1 : xbsIndex_r4/Slice  nbits=W-NB  boolean_output=off  mode=Lower Bit Location + Width  bit1=0  base1=MSB of Input  bit0=0  base0=LSB of Input  dbl_ovrd=off  block_type=slice
  O : Outport
  wires:
  I/1 -> Slice1/1, Slice/1
  Concat/1 -> O/1
  Slice/1 -> Concat/2
  Slice1/1 -> Concat/1

== system XMC_FFT2D_HDL_AIE/hdl_2dfft/Read BarrelShifter/RotateLeft13 ==
  I : Inport
  Concat : xbsIndex_r4/Concat  num_inputs=2  dbl_ovrd=off  block_type=concat
  Slice : xbsIndex_r4/Slice  nbits=NB  boolean_output=off  mode=Upper Bit Location + Width  bit1=0  base1=MSB of Input  bit0=0  base0=LSB of Input  dbl_ovrd=off  block_type=slice
  Slice1 : xbsIndex_r4/Slice  nbits=W-NB  boolean_output=off  mode=Lower Bit Location + Width  bit1=0  base1=MSB of Input  bit0=0  base0=LSB of Input  dbl_ovrd=off  block_type=slice
  O : Outport
  wires:
  I/1 -> Slice1/1, Slice/1
  Concat/1 -> O/1
  Slice/1 -> Concat/2
  Slice1/1 -> Concat/1

== system XMC_FFT2D_HDL_AIE/hdl_2dfft/Read BarrelShifter/RotateLeft14 ==
  I : Inport
  Concat : xbsIndex_r4/Concat  num_inputs=2  dbl_ovrd=off  block_type=concat
  Slice : xbsIndex_r4/Slice  nbits=NB  boolean_output=off  mode=Upper Bit Location + Width  bit1=0  base1=MSB of Input  bit0=0  base0=LSB of Input  dbl_ovrd=off  block_type=slice
  Slice1 : xbsIndex_r4/Slice  nbits=W-NB  boolean_output=off  mode=Lower Bit Location + Width  bit1=0  base1=MSB of Input  bit0=0  base0=LSB of Input  dbl_ovrd=off  block_type=slice
  O : Outport
  wires:
  I/1 -> Slice1/1, Slice/1
  Concat/1 -> O/1
  Slice/1 -> Concat/2
  Slice1/1 -> Concat/1

== system XMC_FFT2D_HDL_AIE/hdl_2dfft/Read BarrelShifter/RotateLeft15 ==
  I : Inport
  Concat : xbsIndex_r4/Concat  num_inputs=2  dbl_ovrd=off  block_type=concat
  Slice : xbsIndex_r4/Slice  nbits=NB  boolean_output=off  mode=Upper Bit Location + Width  bit1=0  base1=MSB of Input  bit0=0  base0=LSB of Input  dbl_ovrd=off  block_type=slice
  Slice1 : xbsIndex_r4/Slice  nbits=W-NB  boolean_output=off  mode=Lower Bit Location + Width  bit1=0  base1=MSB of Input  bit0=0  base0=LSB of Input  dbl_ovrd=off  block_type=slice
  O : Outport
  wires:
  I/1 -> Slice1/1, Slice/1
  Concat/1 -> O/1
  Slice/1 -> Concat/2
  Slice1/1 -> Concat/1

== system XMC_FFT2D_HDL_AIE/hdl_2dfft/Read BarrelShifter/RotateLeft2 ==
  I : Inport
  Concat : xbsIndex_r4/Concat  num_inputs=2  dbl_ovrd=off  block_type=concat
  Slice : xbsIndex_r4/Slice  nbits=NB  boolean_output=off  mode=Upper Bit Location + Width  bit1=0  base1=MSB of Input  bit0=0  base0=LSB of Input  dbl_ovrd=off  block_type=slice
  Slice1 : xbsIndex_r4/Slice  nbits=W-NB  boolean_output=off  mode=Lower Bit Location + Width  bit1=0  base1=MSB of Input  bit0=0  base0=LSB of Input  dbl_ovrd=off  block_type=slice
  O : Outport
  wires:
  I/1 -> Slice1/1, Slice/1
  Concat/1 -> O/1
  Slice/1 -> Concat/2
  Slice1/1 -> Concat/1

== system XMC_FFT2D_HDL_AIE/hdl_2dfft/Read BarrelShifter/RotateLeft3 ==
  I : Inport
  Concat : xbsIndex_r4/Concat  num_inputs=2  dbl_ovrd=off  block_type=concat
  Slice : xbsIndex_r4/Slice  nbits=NB  boolean_output=off  mode=Upper Bit Location + Width  bit1=0  base1=MSB of Input  bit0=0  base0=LSB of Input  dbl_ovrd=off  block_type=slice
  Slice1 : xbsIndex_r4/Slice  nbits=W-NB  boolean_output=off  mode=Lower Bit Location + Width  bit1=0  base1=MSB of Input  bit0=0  base0=LSB of Input  dbl_ovrd=off  block_type=slice
  O : Outport
  wires:
  I/1 -> Slice1/1, Slice/1
  Concat/1 -> O/1
  Slice/1 -> Concat/2
  Slice1/1 -> Concat/1

== system XMC_FFT2D_HDL_AIE/hdl_2dfft/Read BarrelShifter/RotateLeft4 ==
  I : Inport
  Concat : xbsIndex_r4/Concat  num_inputs=2  dbl_ovrd=off  block_type=concat
  Slice : xbsIndex_r4/Slice  nbits=NB  boolean_output=off  mode=Upper Bit Location + Width  bit1=0  base1=MSB of Input  bit0=0  base0=LSB of Input  dbl_ovrd=off  block_type=slice
  Slice1 : xbsIndex_r4/Slice  nbits=W-NB  boolean_output=off  mode=Lower Bit Location + Width  bit1=0  base1=MSB of Input  bit0=0  base0=LSB of Input  dbl_ovrd=off  block_type=slice
  O : Outport
  wires:
  I/1 -> Slice1/1, Slice/1
  Concat/1 -> O/1
  Slice/1 -> Concat/2
  Slice1/1 -> Concat/1

== system XMC_FFT2D_HDL_AIE/hdl_2dfft/Read BarrelShifter/RotateLeft5 ==
  I : Inport
  Concat : xbsIndex_r4/Concat  num_inputs=2  dbl_ovrd=off  block_type=concat
  Slice : xbsIndex_r4/Slice  nbits=NB  boolean_output=off  mode=Upper Bit Location + Width  bit1=0  base1=MSB of Input  bit0=0  base0=LSB of Input  dbl_ovrd=off  block_type=slice
  Slice1 : xbsIndex_r4/Slice  nbits=W-NB  boolean_output=off  mode=Lower Bit Location + Width  bit1=0  base1=MSB of Input  bit0=0  base0=LSB of Input  dbl_ovrd=off  block_type=slice
  O : Outport
  wires:
  I/1 -> Slice1/1, Slice/1
  Concat/1 -> O/1
  Slice/1 -> Concat/2
  Slice1/1 -> Concat/1

== system XMC_FFT2D_HDL_AIE/hdl_2dfft/Read BarrelShifter/RotateLeft6 ==
  I : Inport
  Concat : xbsIndex_r4/Concat  num_inputs=2  dbl_ovrd=off  block_type=concat
  Slice : xbsIndex_r4/Slice  nbits=NB  boolean_output=off  mode=Upper Bit Location + Width  bit1=0  base1=MSB of Input  bit0=0  base0=LSB of Input  dbl_ovrd=off  block_type=slice
  Slice1 : xbsIndex_r4/Slice  nbits=W-NB  boolean_output=off  mode=Lower Bit Location + Width  bit1=0  base1=MSB of Input  bit0=0  base0=LSB of Input  dbl_ovrd=off  block_type=slice
  O : Outport
  wires:
  I/1 -> Slice1/1, Slice/1
  Concat/1 -> O/1
  Slice/1 -> Concat/2
  Slice1/1 -> Concat/1

== system XMC_FFT2D_HDL_AIE/hdl_2dfft/Read BarrelShifter/RotateLeft7 ==
  I : Inport
  Concat : xbsIndex_r4/Concat  num_inputs=2  dbl_ovrd=off  block_type=concat
  Slice : xbsIndex_r4/Slice  nbits=NB  boolean_output=off  mode=Upper Bit Location + Width  bit1=0  base1=MSB of Input  bit0=0  base0=LSB of Input  dbl_ovrd=off  block_type=slice
  Slice1 : xbsIndex_r4/Slice  nbits=W-NB  boolean_output=off  mode=Lower Bit Location + Width  bit1=0  base1=MSB of Input  bit0=0  base0=LSB of Input  dbl_ovrd=off  block_type=slice
  O : Outport
  wires:
  I/1 -> Slice1/1, Slice/1
  Concat/1 -> O/1
  Slice/1 -> Concat/2
  Slice1/1 -> Concat/1

== system XMC_FFT2D_HDL_AIE/hdl_2dfft/Read BarrelShifter/RotateLeft8 ==
  I : Inport
  Concat : xbsIndex_r4/Concat  num_inputs=2  dbl_ovrd=off  block_type=concat
  Slice : xbsIndex_r4/Slice  nbits=NB  boolean_output=off  mode=Upper Bit Location + Width  bit1=0  base1=MSB of Input  bit0=0  base0=LSB of Input  dbl_ovrd=off  block_type=slice
  Slice1 : xbsIndex_r4/Slice  nbits=W-NB  boolean_output=off  mode=Lower Bit Location + Width  bit1=0  base1=MSB of Input  bit0=0  base0=LSB of Input  dbl_ovrd=off  block_type=slice
  O : Outport
  wires:
  I/1 -> Slice1/1, Slice/1
  Concat/1 -> O/1
  Slice/1 -> Concat/2
  Slice1/1 -> Concat/1

== system XMC_FFT2D_HDL_AIE/hdl_2dfft/Read BarrelShifter/RotateLeft9 ==
  I : Inport
  Concat : xbsIndex_r4/Concat  num_inputs=2  dbl_ovrd=off  block_type=concat
  Slice : xbsIndex_r4/Slice  nbits=NB  boolean_output=off  mode=Upper Bit Location + Width  bit1=0  base1=MSB of Input  bit0=0  base0=LSB of Input  dbl_ovrd=off  block_type=slice
  Slice1 : xbsIndex_r4/Slice  nbits=W-NB  boolean_output=off  mode=Lower Bit Location + Width  bit1=0  base1=MSB of Input  bit0=0  base0=LSB of Input  dbl_ovrd=off  block_type=slice
  O : Outport
  wires:
  I/1 -> Slice1/1, Slice/1
  Concat/1 -> O/1
  Slice/1 -> Concat/2
  Slice1/1 -> Concat/1

== system XMC_FFT2D_HDL_AIE/hdl_2dfft/Write BarrelShifter/RotateLeft1 ==
  I : Inport
  Concat : xbsIndex_r4/Concat  num_inputs=2  dbl_ovrd=off  block_type=concat
  Slice : xbsIndex_r4/Slice  nbits=NB  boolean_output=off  mode=Upper Bit Location + Width  bit1=0  base1=MSB of Input  bit0=0  base0=LSB of Input  dbl_ovrd=off  block_type=slice
  Slice1 : xbsIndex_r4/Slice  nbits=W-NB  boolean_output=off  mode=Lower Bit Location + Width  bit1=0  base1=MSB of Input  bit0=0  base0=LSB of Input  dbl_ovrd=off  block_type=slice
  O : Outport
  wires:
  I/1 -> Slice1/1, Slice/1
  Concat/1 -> O/1
  Slice/1 -> Concat/2
  Slice1/1 -> Concat/1

== system XMC_FFT2D_HDL_AIE/hdl_2dfft/Write BarrelShifter/RotateLeft10 ==
  I : Inport
  Concat : xbsIndex_r4/Concat  num_inputs=2  dbl_ovrd=off  block_type=concat
  Slice : xbsIndex_r4/Slice  nbits=NB  boolean_output=off  mode=Upper Bit Location + Width  bit1=0  base1=MSB of Input  bit0=0  base0=LSB of Input  dbl_ovrd=off  block_type=slice
  Slice1 : xbsIndex_r4/Slice  nbits=W-NB  boolean_output=off  mode=Lower Bit Location + Width  bit1=0  base1=MSB of Input  bit0=0  base0=LSB of Input  dbl_ovrd=off  block_type=slice
  O : Outport
  wires:
  Slice1/1 -> Concat/1
  Slice/1 -> Concat/2
  Concat/1 -> O/1
  I/1 -> Slice/1, Slice1/1

== system XMC_FFT2D_HDL_AIE/hdl_2dfft/Write BarrelShifter/RotateLeft11 ==
  I : Inport
  Concat : xbsIndex_r4/Concat  num_inputs=2  dbl_ovrd=off  block_type=concat
  Slice : xbsIndex_r4/Slice  nbits=NB  boolean_output=off  mode=Upper Bit Location + Width  bit1=0  base1=MSB of Input  bit0=0  base0=LSB of Input  dbl_ovrd=off  block_type=slice
  Slice1 : xbsIndex_r4/Slice  nbits=W-NB  boolean_output=off  mode=Lower Bit Location + Width  bit1=0  base1=MSB of Input  bit0=0  base0=LSB of Input  dbl_ovrd=off  block_type=slice
  O : Outport
  wires:
  Slice1/1 -> Concat/1
  Slice/1 -> Concat/2
  Concat/1 -> O/1
  I/1 -> Slice/1, Slice1/1

== system XMC_FFT2D_HDL_AIE/hdl_2dfft/Write BarrelShifter/RotateLeft12 ==
  I : Inport
  Concat : xbsIndex_r4/Concat  num_inputs=2  dbl_ovrd=off  block_type=concat
  Slice : xbsIndex_r4/Slice  nbits=NB  boolean_output=off  mode=Upper Bit Location + Width  bit1=0  base1=MSB of Input  bit0=0  base0=LSB of Input  dbl_ovrd=off  block_type=slice
  Slice1 : xbsIndex_r4/Slice  nbits=W-NB  boolean_output=off  mode=Lower Bit Location + Width  bit1=0  base1=MSB of Input  bit0=0  base0=LSB of Input  dbl_ovrd=off  block_type=slice
  O : Outport
  wires:
  Slice1/1 -> Concat/1
  Slice/1 -> Concat/2
  Concat/1 -> O/1
  I/1 -> Slice/1, Slice1/1

== system XMC_FFT2D_HDL_AIE/hdl_2dfft/Write BarrelShifter/RotateLeft13 ==
  I : Inport
  Concat : xbsIndex_r4/Concat  num_inputs=2  dbl_ovrd=off  block_type=concat
  Slice : xbsIndex_r4/Slice  nbits=NB  boolean_output=off  mode=Upper Bit Location + Width  bit1=0  base1=MSB of Input  bit0=0  base0=LSB of Input  dbl_ovrd=off  block_type=slice
  Slice1 : xbsIndex_r4/Slice  nbits=W-NB  boolean_output=off  mode=Lower Bit Location + Width  bit1=0  base1=MSB of Input  bit0=0  base0=LSB of Input  dbl_ovrd=off  block_type=slice
  O : Outport
  wires:
  Slice1/1 -> Concat/1
  Slice/1 -> Concat/2
  Concat/1 -> O/1
  I/1 -> Slice/1, Slice1/1

== system XMC_FFT2D_HDL_AIE/hdl_2dfft/Write BarrelShifter/RotateLeft14 ==
  I : Inport
  Concat : xbsIndex_r4/Concat  num_inputs=2  dbl_ovrd=off  block_type=concat
  Slice : xbsIndex_r4/Slice  nbits=NB  boolean_output=off  mode=Upper Bit Location + Width  bit1=0  base1=MSB of Input  bit0=0  base0=LSB of Input  dbl_ovrd=off  block_type=slice
  Slice1 : xbsIndex_r4/Slice  nbits=W-NB  boolean_output=off  mode=Lower Bit Location + Width  bit1=0  base1=MSB of Input  bit0=0  base0=LSB of Input  dbl_ovrd=off  block_type=slice
  O : Outport
  wires:
  Slice1/1 -> Concat/1
  Slice/1 -> Concat/2
  Concat/1 -> O/1
  I/1 -> Slice/1, Slice1/1

== system XMC_FFT2D_HDL_AIE/hdl_2dfft/Write BarrelShifter/RotateLeft15 ==
  I : Inport
  Concat : xbsIndex_r4/Concat  num_inputs=2  dbl_ovrd=off  block_type=concat
  Slice : xbsIndex_r4/Slice  nbits=NB  boolean_output=off  mode=Upper Bit Location + Width  bit1=0  base1=MSB of Input  bit0=0  base0=LSB of Input  dbl_ovrd=off  block_type=slice
  Slice1 : xbsIndex_r4/Slice  nbits=W-NB  boolean_output=off  mode=Lower Bit Location + Width  bit1=0  base1=MSB of Input  bit0=0  base0=LSB of Input  dbl_ovrd=off  block_type=slice
  O : Outport
  wires:
  Slice1/1 -> Concat/1
  Slice/1 -> Concat/2
  Concat/1 -> O/1
  I/1 -> Slice/1, Slice1/1

== system XMC_FFT2D_HDL_AIE/hdl_2dfft/Write BarrelShifter/RotateLeft2 ==
  I : Inport
  Concat : xbsIndex_r4/Concat  num_inputs=2  dbl_ovrd=off  block_type=concat
  Slice : xbsIndex_r4/Slice  nbits=NB  boolean_output=off  mode=Upper Bit Location + Width  bit1=0  base1=MSB of Input  bit0=0  base0=LSB of Input  dbl_ovrd=off  block_type=slice
  Slice1 : xbsIndex_r4/Slice  nbits=W-NB  boolean_output=off  mode=Lower Bit Location + Width  bit1=0  base1=MSB of Input  bit0=0  base0=LSB of Input  dbl_ovrd=off  block_type=slice
  O : Outport
  wires:
  Slice1/1 -> Concat/1
  Slice/1 -> Concat/2
  Concat/1 -> O/1
  I/1 -> Slice/1, Slice1/1
